simulink model "MOTOR_DC"  (R2018a)
settings: Solver=VariableStepAuto  StartTime=0.0  StopTime=3  RelTol=1e-3
values from neighbouring files (symbols this model uses):
  b = 3.5077e-06    [Prj_7.m]
  J = 3.2284e-04    (= 0.00032284)    [Prj_7.m]
  Kb = 0.0274    [Prj_7.m]
  Kt = 0.0274    [Prj_7.m]
  L = 2.75e-06    [Prj_7.m]
  R = 4    [Prj_7.m]
libraries: simulink x1
settings Model: Creator=Dpt_Mas  LastModifiedBy=Dpt_Mas

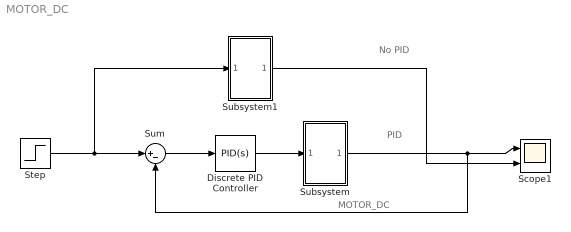
== system MOTOR_DC ==
  note: PID
  note: No PID
  note: MOTOR_DC
  Discrete PID Controller : simulink/Continuous/PID Controller  Controller=PID  TimeDomain=Continuous-time  SampleTime=-1  IntegratorMethod=Forward Euler  FilterMethod=Forward Euler  Form=Parallel  UseFilter=on  ControllerParametersSource=internal  P=3  I=1  D=0.01  N=100  InitialConditionSource=internal  InitialConditionForIntegrator=0  InitialConditionForFilter=0  ExternalReset=none  LimitOutput=off  UpperSaturationLimit=inf  LowerSaturationLimit=-inf  LinearizeAsGain=off  AntiWindupMode=none  Kb=1  TrackingMode=off  Kt=1  PParamMin=[]  PParamMax=[]  IParamMin=[]  IParamMax=[]  DParamMin=[]  DParamMax=[]  NParamMin=[]  NParamMax=[]  KbParamMin=[]  KbParamMax=[]  KtParamMin=[]  KtParamMax=[]  POutMin=[]  POutMax=[]  IOutMin=[]  IOutMax=[]  DOutMin=[]  DOutMax=[]  NOutMin=[]  NOutMax=[]  KbOutMin=[]  KbOutMax=[]  KtOutMin=[]  KtOutMax=[]  IntegratorOutMin=[]  IntegratorOutMax=[]  FilterOutMin=[]  FilterOutMax=[]  SumOutMin=[]  SumOutMax=[]  SumI1OutMin=[]  SumI1OutMax=[]  SumI2OutMin=[]  SumI2OutMax=[]  SumI3OutMin=[]  SumI3OutMax=[]  SumDOutMin=[]  SumDOutMax=[]  SaturationOutMin=[]  SaturationOutMax=[]  IntegratorContinuousStateAttributes=''  IntegratorStateMustResolveToSignalObject=off  IntegratorRTWStateStorageClass=Auto  FilterContinuousStateAttributes=''  FilterStateMustResolveToSignalObject=off  FilterRTWStateStorageClass=Auto  DifferentiatorICPrevScaledInput=0  DifferentiatorOutMin=[]  DifferentiatorOutMax=[]  FilterDiffOutCoefMin=[]  FilterDiffOutCoefMax=[]  SumDenOutMin=[]  SumDenOutMax=[]  SumNumOutMin=[]  SumNumOutMax=[]  ReciprocalOutMin=[]  ReciprocalOutMax=[]  DivideOutMin=[]  DivideOutMax=[]  TunerSelectOption=Transfer Function Based (PID Tuner App)
  Scope1 : Scope  NumInputPorts=2
  Step : Step  SampleTime=0
  Subsystem : Subsystem
  Subsystem1 : Subsystem
  Sum : Sum  Inputs=|+-
  wires:
  Subsystem/1(Out1) -> Scope1/1, Sum/2
  Discrete PID Controller/1 -> Subsystem/1(In1)
  Step/1 -> Subsystem1/1(In1), Sum/1
  Sum/1 -> Discrete PID Controller/1
  Subsystem1/1(Out1) -> Scope1/2

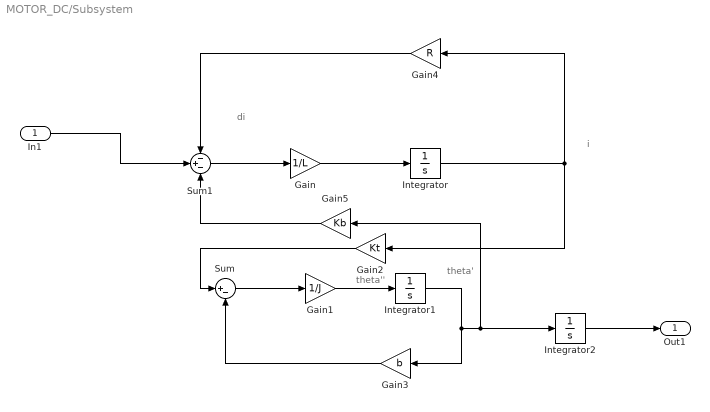
== system MOTOR_DC/Subsystem ==
  note: theta'
  note: theta''
  note: i
  note: di
  In1 : Inport
  Gain : Gain  Gain=1/L
  Gain1 : Gain  Gain=1/J
  Gain2 : Gain  Gain=Kt
  Gain3 : Gain  Gain=b
  Gain4 : Gain  Gain=R
  Gain5 : Gain  Gain=Kb
  Integrator : Integrator
  Integrator1 : Integrator
  Integrator2 : Integrator
  Sum : Sum  Inputs=|+-
  Sum1 : Sum  Inputs=-+-
  Out1 : Outport
  wires:
  Sum/1 -> Gain1/1
  Gain/1 -> Integrator/1
  Integrator1/1 -> Gain5/1, Integrator2/1, Gain3/1
  Gain5/1 -> Sum1/3
  Integrator/1 -> Gain2/1, Gain4/1
  Sum1/1 -> Gain/1
  Gain2/1 -> Sum/1
  Gain3/1 -> Sum/2
  Gain1/1 -> Integrator1/1
  Integrator2/1 -> Out1/1
  Gain4/1 -> Sum1/1
  In1/1 -> Sum1/2

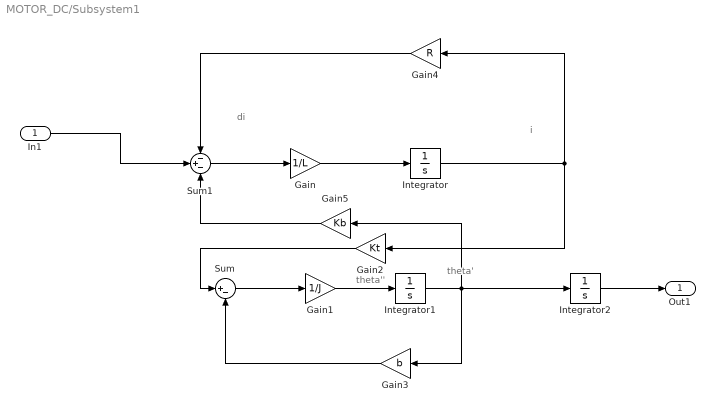
== system MOTOR_DC/Subsystem1 ==
  note: di
  note: i
  note: theta''
  note: theta'
  In1 : Inport
  Gain : Gain  Gain=1/L
  Gain1 : Gain  Gain=1/J
  Gain2 : Gain  Gain=Kt
  Gain3 : Gain  Gain=b
  Gain4 : Gain  Gain=R
  Gain5 : Gain  Gain=Kb
  Integrator : Integrator
  Integrator1 : Integrator
  Integrator2 : Integrator
  Sum : Sum  Inputs=|+-
  Sum1 : Sum  Inputs=-+-
  Out1 : Outport
  wires:
  In1/1 -> Sum1/2
  Gain4/1 -> Sum1/1
  Integrator2/1 -> Out1/1
  Gain1/1 -> Integrator1/1
  Gain3/1 -> Sum/2
  Gain2/1 -> Sum/1
  Sum1/1 -> Gain/1
  Integrator/1 -> Gain4/1, Gain2/1
  Gain5/1 -> Sum1/3
  Integrator1/1 -> Gain3/1, Integrator2/1, Gain5/1
  Gain/1 -> Integrator/1
  Sum/1 -> Gain1/1
